simulink model "untitled"  (R2017a)
settings: Solver=VariableStepAuto  StartTime=0.0  StopTime=10.0  MaxStep=1e-4  RelTol=1e-3
libraries: simulink_extras x3, powerlib x1
settings Model: Creator=Usama Abbas  LastModifiedBy=Usama Abbas

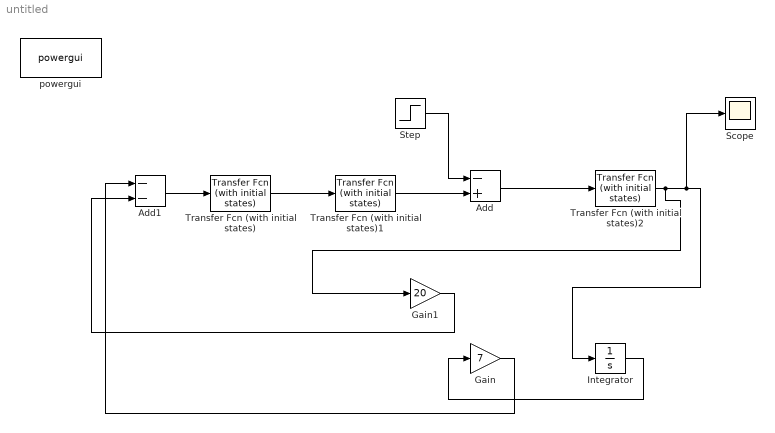
== system untitled ==
  Add : Sum  Inputs=-+
  Add1 : Sum  Inputs=--
  Gain : Gain  Gain=7
  Gain1 : Gain  Gain=20
  Integrator : Integrator
  Scope : Scope
  Step : Step  SampleTime=0
  Transfer Fcn (with initial states) : simulink_extras/Additional Linear/Transfer Fcn (with initial states)  N=[1]  D="[0.2  1]"  X0=.5
  Transfer Fcn (with initial states)1 : simulink_extras/Additional Linear/Transfer Fcn (with initial states)  N=[1]  D="[0.5  1]"  X0=.5
  Transfer Fcn (with initial states)2 : simulink_extras/Additional Linear/Transfer Fcn (with initial states)  N=[1]  D="[10  0.5]"  X0=.5
  powergui : powerlib/powergui  Priority=1  SimulationMode=Continuous  SampleTime=50e-6  frequency=60  Iterations=50  frequencyindice=60  Pbase=100e6  ErrMax=1e-4  UnitsV=kV  UnitsW=MW  buscounter=0  FunctionMessages=off  echomessages=off  EnableUseOfTLC=off  CurrentSourceSwitches=off  DisableSnubberDevices=off  DisableRonSwitches=off  DisableVfSwitches=off  DisplayEquations=off  SolverType=Tustin/Backward Euler (TBE)  Interpol=off  ExternalGateDelay=off  methode=off  Ts=100  x0status=blocks  SPID=on  SwTol=0  HookPort=off  RestoreLinks=warning  ResistiveCurrentMeasurement=off  Frange=[0:2:500]  Ylog=off  Xlog=on  ShowGrid=off  save=off  variable=ZData  structure=0  ZoomFFT=off  StartTime=0.0  cycles=1  DisplayStyle=1  fundamental=60  FreqAxis=off  MaxFrequency=1000  frequencyindicesteady=1  RmsSteady=1  display=off
  wires:
  Add1/1 -> Transfer Fcn (with initial states)/1
  Transfer Fcn (with initial states)/1 -> Transfer Fcn (with initial states)1/1
  Add/1 -> Transfer Fcn (with initial states)2/1
  Transfer Fcn (with initial states)1/1 -> Add/2
  Step/1 -> Add/1
  Transfer Fcn (with initial states)2/1 -> Gain1/1, Scope/1, Integrator/1
  Integrator/1 -> Gain/1
  Gain/1 -> Add1/1
  Gain1/1 -> Add1/2
